simulink model "ProgrammerCalc"  (R2016a)
settings: Solver=FixedStepDiscrete  StartTime=0.0  StopTime=10.0  RelTol=1e-3
model workspace (MAT data in the model file):
  cs : Simulink.ConfigSet (value not decoded)
libraries: simulink x5
settings Model: Creator=LEGION  LastModifiedBy=LEGION
settings OptimizationCC: DefaultParameterBehavior=Inlined  OptimizeModelRefInitCode=on  LifeSpan=1
settings RTWCC: SystemTargetFile=ert.tlc  GenCodeOnly=on  TemplateMakefile=ert_default_tmf  GenerateReport=on  IncludeHyperlinkInReport=on  LaunchReport=on  GenerateTraceInfo=on  GenerateTraceReport=on  GenerateTraceReportSl=on  GenerateTraceReportSf=on  GenerateTraceReportEml=on
settings CodeAppCC: ForceParamTrailComments=on  IgnoreCustomStorageClasses=off  OperatorAnnotations=on  SimulinkDataObjDesc=on  SFDataObjDesc=on  MATLABFcnDesc=on  InsertBlockDesc=on  MATLABSourceComments=on
settings ERTTargetCC: GenerateSampleERTMain=on  InlinedParameterPlacement=NonHierarchical  ERTCustomFileTemplate=example_file_process.tlc

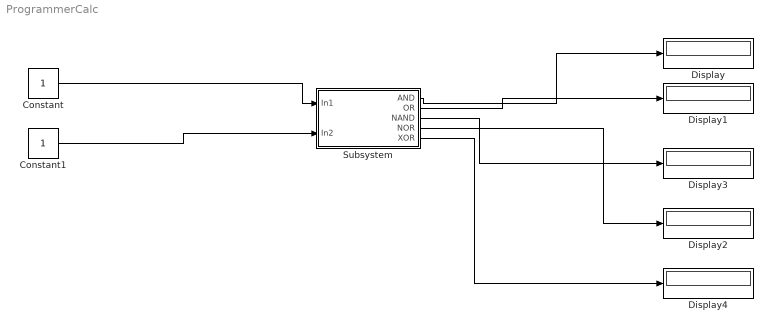
== system ProgrammerCalc ==
  Constant : Constant  OutDataTypeStr=uint8
  Constant1 : Constant  OutDataTypeStr=uint8
  Display{,1..4} (5 alike) : Display
  Subsystem : Subsystem
  wires:
  Subsystem/1(AND) -> Display/1
  Subsystem/2(OR) -> Display1/1
  Subsystem/4(NOR) -> Display2/1
  Subsystem/3(NAND) -> Display3/1
  Subsystem/5(XOR) -> Display4/1
  Constant/1 -> Subsystem/1(In1)
  Constant1/1 -> Subsystem/2(In2)

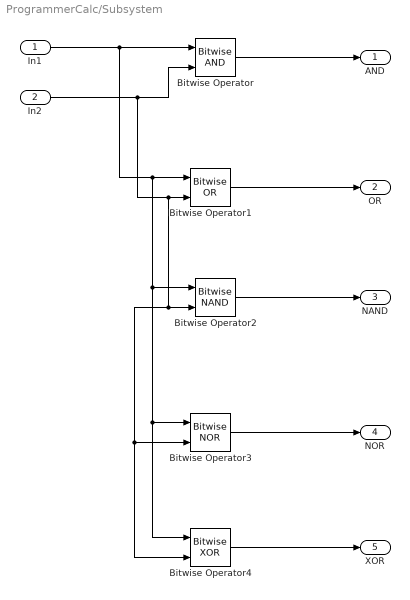
== system ProgrammerCalc/Subsystem ==
  In1 : Inport  OutDataTypeStr=uint8
  In2 : Inport  Port=2  OutDataTypeStr=uint8
  Bitwise Operator : simulink/Logic and Bit Operations/Bitwise Operator  logicop=AND  UseBitMask=off  NumInputPorts=2  BitMask=bin2dec('11011001')  BitMaskRealWorld=Stored Integer
  Bitwise Operator1 : simulink/Logic and Bit Operations/Bitwise Operator  logicop=OR  UseBitMask=off  NumInputPorts=2  BitMask=bin2dec('11011001')  BitMaskRealWorld=Stored Integer
  Bitwise Operator2 : simulink/Logic and Bit Operations/Bitwise Operator  logicop=NAND  UseBitMask=off  NumInputPorts=2  BitMask=bin2dec('11011001')  BitMaskRealWorld=Stored Integer
  Bitwise Operator3 : simulink/Logic and Bit Operations/Bitwise Operator  logicop=NOR  UseBitMask=off  NumInputPorts=2  BitMask=bin2dec('11011001')  BitMaskRealWorld=Stored Integer
  Bitwise Operator4 : simulink/Logic and Bit Operations/Bitwise Operator  logicop=XOR  UseBitMask=off  NumInputPorts=2  BitMask=bin2dec('11011001')  BitMaskRealWorld=Stored Integer
  AND : Outport
  OR : Outport  Port=2
  NAND : Outport  Port=3
  NOR : Outport  Port=4
  XOR : Outport  Port=5
  wires:
  In1/1 -> Bitwise Operator4/1, Bitwise Operator3/1, Bitwise Operator2/1, Bitwise Operator1/1, Bitwise Operator/1
  In2/1 -> Bitwise Operator2/2, Bitwise Operator4/2, Bitwise Operator3/2, Bitwise Operator1/2, Bitwise Operator/2
  Bitwise Operator/1 -> AND/1
  Bitwise Operator1/1 -> OR/1
  Bitwise Operator2/1 -> NAND/1
  Bitwise Operator3/1 -> NOR/1
  Bitwise Operator4/1 -> XOR/1
